simulink model "model4_data"  (R2019b)
settings: Solver=VariableStepAuto  StartTime=0.0  StopTime=15*3600  RelTol=1e-3
PreLoadFcn:
  | % Set physical parameters
  | panelMotorParams;
  | 
  | % Load sun position data for tracking
  | load sunPositionData;
values from neighbouring files (symbols this model uses):
  J = m/12*(l^2*cos(beta)^2+d^2*sin(beta)^2+w^2)    [panelMotorParams.m]
  Kd = 5    [panelMotorParams.m]
  Kf = 0.07    [panelMotorParams.m]
  Kg = 2000    [panelMotorParams.m]
  Kt = 0.07    [panelMotorParams.m]
  L = 1e-5    (= 1e-05)    [panelMotorParams.m]
  R = 10    [panelMotorParams.m]
libraries: simulink x1
settings Model: Creator=bneiswan  LastModifiedBy=bneiswan
settings DataIOCC: ExternalInput=[sunTime,sunPosition]  LoadExternalInput=on

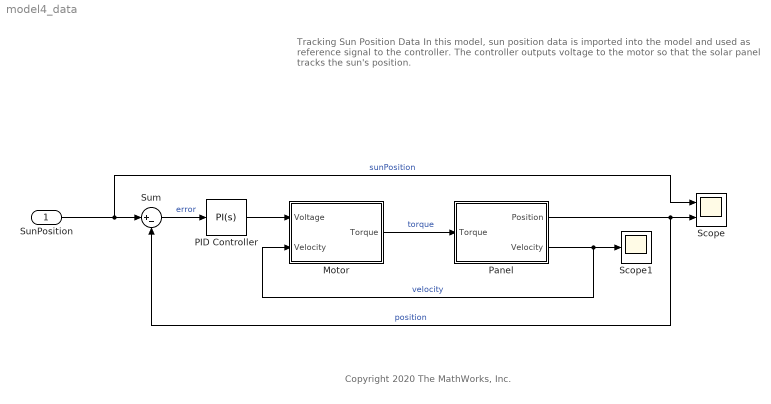
== system model4_data ==
  note: Copyright 2020 The MathWorks, Inc.
  note: Tracking Sun Position Data
      |
      | In this model, sun position data is imported into the model and used as reference signal to the controller. The controller outputs voltage to the motor so that the solar panel tracks the sun's position.
  SunPosition : Inport
  Motor : Subsystem
  PID Controller : simulink/Continuous/PID Controller  Controller=PI  Form=Parallel  TimeDomain=Continuous-time  SampleTime=-1  IntegratorMethod=Forward Euler  FilterMethod=Forward Euler  ControllerParametersSource=internal  P=240  I=180  D=0  UseFilter=on  N=100  TunerSelectOption=Transfer Function Based (PID Tuner App)  InitialConditionSource=internal  InitialConditionForIntegrator=0  InitialConditionForFilter=0  DifferentiatorICPrevScaledInput=0  ExternalReset=none  TrackingMode=off  Kt=1  LimitOutput=off  UpperSaturationLimit=inf  LowerSaturationLimit=-inf  LinearizeAsGain=on  AntiWindupMode=none  Kb=1  POutMin=[]  POutMax=[]  IOutMin=[]  IOutMax=[]  DOutMin=[]  DOutMax=[]  NOutMin=[]  NOutMax=[]  SumOutMin=[]  SumOutMax=[]  SaturationOutMin=[]  SaturationOutMax=[]  PParamMin=[]  PParamMax=[]  IParamMin=[]  IParamMax=[]  DParamMin=[]  DParamMax=[]  NParamMin=[]  NParamMax=[]  KbParamMin=[]  KbParamMax=[]  KtParamMin=[]  KtParamMax=[]  KbOutMin=[]  KbOutMax=[]  KtOutMin=[]  KtOutMax=[]  IntegratorOutMin=[]  IntegratorOutMax=[]  FilterOutMin=[]  FilterOutMax=[]  SumI1OutMin=[]  SumI1OutMax=[]  SumI2OutMin=[]  SumI2OutMax=[]  SumI3OutMin=[]  SumI3OutMax=[]  SumI4OutMin=[]  SumI4OutMax=[]  SumDOutMin=[]  SumDOutMax=[]  DifferentiatorOutMin=[]  DifferentiatorOutMax=[]  FilterDiffOutCoefMin=[]  FilterDiffOutCoefMax=[]  ReciprocalOutMin=[]  ReciprocalOutMax=[]  SumDenOutMin=[]  SumDenOutMax=[]  SumNumOutMin=[]  SumNumOutMax=[]  DivideOutMin=[]  DivideOutMax=[]  IntegratorContinuousStateAttributes=''  IntegratorStateMustResolveToSignalObject=off  IntegratorRTWStateStorageClass=Auto  FilterContinuousStateAttributes=''  FilterStateMustResolveToSignalObject=off  FilterRTWStateStorageClass=Auto  ParallelPVariant=InternalParameters  IdealPVariant=Disabled  IVariant=InternalParameters  DVariant=Disabled  IntegratorVariant=Continuous  SatVariant=Disabled  AWVariant=Passthrough  PCopyVariant=Disabled  TRVariant=Disabled  FdbkBlocksVariant=Forward  IdealPFdbkVariant=Disabled  SatFdbkVariant=Disabled  DerivativeFilterVariant=Disabled  NVariant=Disabled  NCopyVariant=Disabled_SignalSpec  FilterICVariant=Disabled  IntegratorICVariant=InternalICs  ExternalResetVariant=Disabled  TRSumVariant=Passthrough  SumFdbkVariant=Disabled  SumVariant=Sum_PI
  Panel : Subsystem
  Scope : Scope  NumInputPorts=2
  Scope1 : Scope
  Sum : Sum  Inputs=|+-
  wires:
  Panel/1(Position) -> Scope/2, Sum/2  "position"
  Motor/1(Torque) -> Panel/1(Torque)  "torque"
  Sum/1 -> PID Controller/1  "error"
  PID Controller/1 -> Motor/1(Voltage)
  Panel/2(Velocity) -> Motor/2(Velocity), Scope1/1  "velocity"
  SunPosition/1 -> Sum/1, Scope/1  "sunPosition"

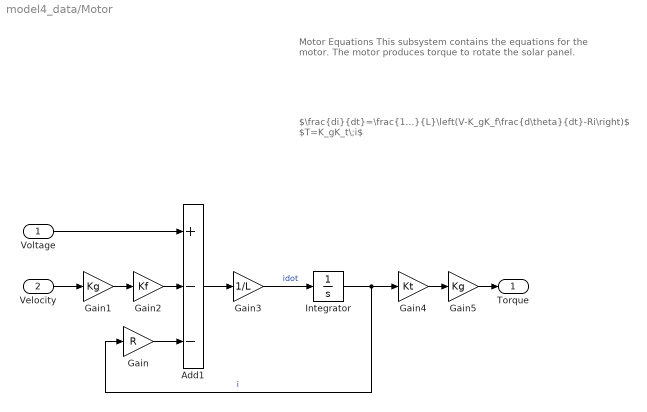
== system model4_data/Motor ==
  note: $\frac{di}{dt}=\frac{1}{L}\left(V-K_gK_f\frac{d\theta}{dt}-Ri\right)$
      | $T=K_gK_t\;i$
  note: Motor Equations
      |
      | This subsystem contains the equations for the motor. The motor produces torque to rotate the solar panel.
  Voltage : Inport
  Velocity : Inport  Port=2
  Add1 : Sum  Inputs=+--
  Gain : Gain  Gain=R
  Gain1 : Gain  Gain=Kg
  Gain2 : Gain  Gain=Kf
  Gain3 : Gain  Gain=1/L
  Gain4 : Gain  Gain=Kt
  Gain5 : Gain  Gain=Kg
  Integrator : Integrator
  Torque : Outport
  wires:
  Voltage/1 -> Add1/1
  Gain2/1 -> Add1/2
  Gain3/1 -> Integrator/1  "idot"
  Gain/1 -> Add1/3
  Integrator/1 -> Gain4/1, Gain/1  "i"
  Add1/1 -> Gain3/1
  Velocity/1 -> Gain1/1
  Gain4/1 -> Gain5/1
  Gain1/1 -> Gain2/1
  Gain5/1 -> Torque/1

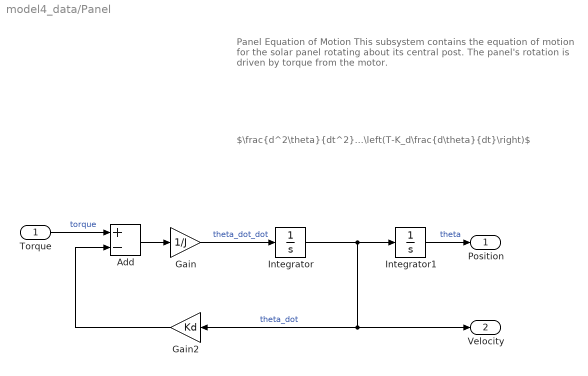
== system model4_data/Panel ==
  note: $\frac{d^2\theta}{dt^2}=\frac{1}{J}\left(T-K_d\frac{d\theta}{dt}\right)$
  note: Panel Equation of Motion
      |
      | This subsystem contains the equation of motion for the solar panel rotating about its central post. The panel's rotation is driven by torque from the motor.
  Torque : Inport
  Add : Sum  Inputs=+-
  Gain : Gain  Gain=1/J
  Gain2 : Gain  Gain=Kd
  Integrator : Integrator
  Integrator1 : Integrator
  Position : Outport
  Velocity : Outport  Port=2
  wires:
  Torque/1 -> Add/1  "torque"
  Add/1 -> Gain/1
  Integrator/1 -> Integrator1/1, Velocity/1, Gain2/1  "theta_dot"
  Gain2/1 -> Add/2
  Gain/1 -> Integrator/1  "theta_dot_dot"
  Integrator1/1 -> Position/1  "theta"
